simulink model "thermal_storage_tank"  (R2017a)
settings: Solver=VariableStepAuto  StartTime=0.0  StopTime=50000  RelTol=1e-3
settings Model: Creator=info  LastModifiedBy=info

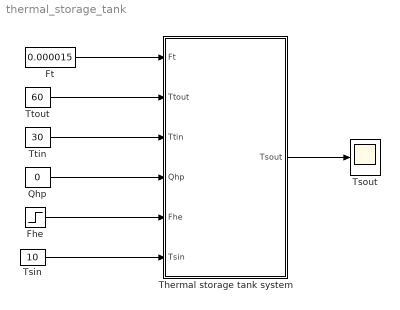
== system thermal_storage_tank ==
  "Fhe " : Step  Time=5  After=0.000015  SampleTime=0
  "Ft " : Constant  Value=0.000015
  Qhp : Constant  Value=0
  Thermal storage tank system : Subsystem
      mask Display: image('storage_tank.PNG');
  Tsin : Constant  Value=10
  Tsout : Scope
  Ttin : Constant  Value=30
  Ttout : Constant  Value=60
  wires:
  Ttin/1 -> Thermal storage tank system/3(Ttin)
  Ttout/1 -> Thermal storage tank system/2("Ttout ")
  "Ft "/1 -> Thermal storage tank system/1("Ft ")
  Thermal storage tank system/1("Tsout ") -> Tsout/1
  "Fhe "/1 -> Thermal storage tank system/5(Fhe)
  Qhp/1 -> Thermal storage tank system/4(Qhp)
  Tsin/1 -> Thermal storage tank system/6(Tsin)

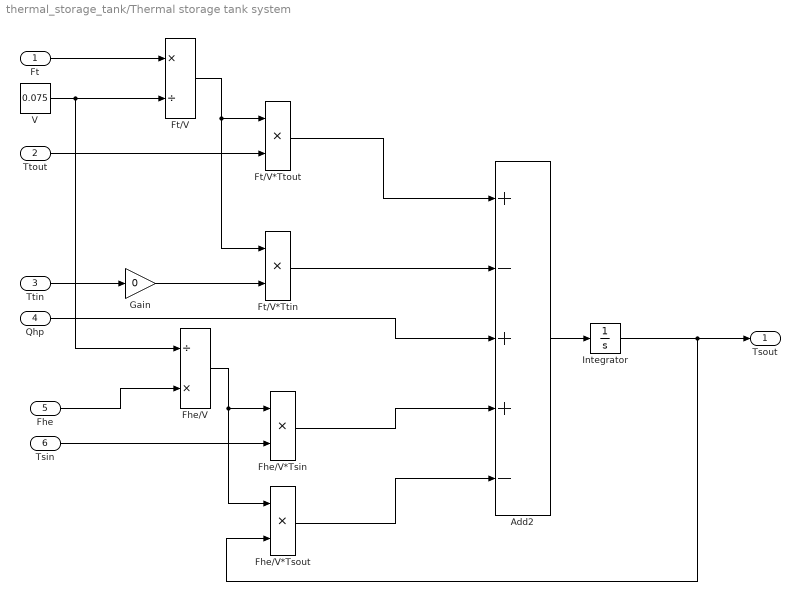
== system thermal_storage_tank/Thermal storage tank system ==
  "Ft " : Inport
  "Ttout " : Inport  Port=2
  Ttin : Inport  Port=3
  Qhp : Inport  Port=4
  Fhe : Inport  Port=5
  Tsin : Inport  Port=6
  Add2 : Sum  Inputs=+-++-
  Fhe/V : Product  Inputs=/*
  Fhe/V*Tsin : Product  Inputs=**
  Fhe/V*Tsout : Product  Inputs=**
  Ft/V : Product  Inputs=*/
  Ft/V*Ttin : Product  Inputs=**
  Ft/V*Ttout : Product  Inputs=**
  Gain : Gain  Gain=0
  Integrator : Integrator  InitialCondition=16.87
  V : Constant  Value=0.075
  "Tsout " : Outport
  wires:
  "Ft "/1 -> Ft/V/1
  Ft/V/1 -> Ft/V*Ttin/1, Ft/V*Ttout/1
  Integrator/1 -> "Tsout "/1, Fhe/V*Tsout/2
  "Ttout "/1 -> Ft/V*Ttout/2
  Ft/V*Ttout/1 -> Add2/1
  Add2/1 -> Integrator/1
  Ft/V*Ttin/1 -> Add2/2
  Ttin/1 -> Gain/1
  Tsin/1 -> Fhe/V*Tsin/2
  Fhe/V/1 -> Fhe/V*Tsout/1, Fhe/V*Tsin/1
  Fhe/V*Tsin/1 -> Add2/4
  V/1 -> Fhe/V/1, Ft/V/2
  Fhe/1 -> Fhe/V/2
  Qhp/1 -> Add2/3
  Fhe/V*Tsout/1 -> Add2/5
  Gain/1 -> Ft/V*Ttin/2
